simulink model "CoVMD_SpdCoord"  (R2016b)
settings: configuration reference "CodeGenConfigSet" (kept outside this file)
settings Model: Creator=lenovo  LastModifiedBy=lenovo
settings ConfigSetRef: SourceLocation=Base Workspace

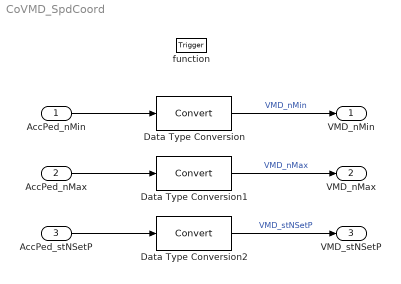
== system CoVMD_SpdCoord ==
  AccPed_nMin : Inport  Tag=rpm  Description=Minimum engine speed in case of accelerator pedal error  OutMin=0  OutMax=6000  OutDataTypeStr=EngSpeed_rpm
  AccPed_nMax : Inport  Tag=rpm  Description=Maximum engine speed in case of accelerator pedal error  Port=2  OutMin=0  OutMax=6000  OutDataTypeStr=EngSpeed_rpm
  AccPed_stNSetP : Inport  Description=Status of engine speed demand of driver demand interpretation  Port=3  OutMin=0  OutMax=255  OutDataTypeStr=State_uint8
  function : TriggerPort  TriggerType=function-call  VariantControl=Variant
  Data Type Conversion : DataTypeConversion
  Data Type Conversion1 : DataTypeConversion
  Data Type Conversion2 : DataTypeConversion
  VMD_nMin : Outport  Tag=rpm  Description=Minimum engine speed limitation after driving assistance coordination  OutMin=-12000  OutMax=12000  OutDataTypeStr=EngSpeed_rpm
  VMD_nMax : Outport  Tag=rpm  Description=Maximum engine speed limitation after driving assistance coordination  Port=2  OutMin=-12000  OutMax=12000  OutDataTypeStr=EngSpeed_rpm
  VMD_stNSetP : Outport  Description=Status of engine speed request after driving assistance coordination  Port=3  OutMin=0  OutMax=255  OutDataTypeStr=State_uint8
  wires:
  Data Type Conversion2/1 -> VMD_stNSetP/1  "VMD_stNSetP"
  Data Type Conversion1/1 -> VMD_nMax/1  "VMD_nMax"
  Data Type Conversion/1 -> VMD_nMin/1  "VMD_nMin"
  AccPed_nMin/1 -> Data Type Conversion/1
  AccPed_nMax/1 -> Data Type Conversion1/1
  AccPed_stNSetP/1 -> Data Type Conversion2/1
